simulink model "ES105A_StHlthSigNormn"  (R2013b)
settings: Solver=FixedStepDiscrete  SolverMode=SingleTasking  StartTime=0.0  StopTime=1  FixedStep=0.002  RelTol=1e-3
undefined symbols (not defined in the file): ARCHGLBPRM_FLOATZEROTHD_ULS_F32, CurrMeasCorrlnMaxErrCurr, CURRMOTSUMDIVBYZEROPROTNVAL_AMPR_F32, DIGTQDIVBYZEROPROTNVAL_HWNWTMTR_F32, DutyCycThermProtnDutyCycFildThd, EcuTMeasRngDiagcMax, EcuTMeasRngDiagcMin, EotLrngAuthyStrtLrn, FRICESTIMNDIVBYZEROPROTNVAL_HWNWTMTR_F32, HLTH0PERC_CNT_U08, HLTH100PERC_CNT_F32, HLTH100PERC_CNT_U08, HLTH50PERC_CNT_U08, HwTqCorrlnChATraSumSetFltThd, HwTqCorrlnChBTraSumSetFltThd, HWTQIDPTSIG_CNT_U08, MOTAG2MEAS_VALMAXERR_VOLTSQD_F32, MOTAG2MEAS_VALMINERR_VOLTSQD_F32, MOTAGCORRLN_MOTAGCORRLNERRTHD_MOTREVELEC_U0P16, MotDrvDiagcErrThd, MOTPOS2DIVBYZEROPROTNVAL2_VOLTSQD_F32, MOTPOS2DIVBYZEROPROTNVAL_VOLTSQD_F32, MOTPOSNERRDIVBYZEROPROTNVAL_MOTREV_U16, MOTPOSNERRZEROTHD_MOTREV_U0P16, NtcNr1, NtcSts1, PHAVLTGDIVBYZEROPROTNVAL_NANOSEC_F32, SigQlfr1, STHLTHSCAGFAC_CNT_F32, StHlthSigNormnAbsltMotPosDifStHlthDiagThd, StHlthSigNormnCurrMotSumStHlthDiagThd, StHlthSigNormnDigTqStHlthDiagThd, StHlthSigNormnDutyCycFltLimThd, StHlthSigNormnHiCtrlrT, StHlthSigNormnIdptSigStHlthSca, StHlthSigNormnLoCtrlrT, StHlthSigNormnMaxFricThd, StHlthSigNormnMinRackTrvlLim, StHlthSigNormnMotPosStHlthDiagThd, StHlthSigNormnMotVelCal, StHlthSigNormnPhaInfoStHlthDiagThd, StHlthSigNormnStHlthCorrlnErr, StHlthSigNormnStHlthCurrMotSum, StHlthSigNormnStHlthPhaInfo, StHlthSigNormnValMaxStHlthErr, StHlthSigNormnValMinStHlthErr, StHlthSigNormnWhlImbRejctnThd, SysGlbPrmMotPoleCnt, TSTHLTH0PERC_CNT_U08, u2, u3, u4, VLTGSTHLTH0PERC_CNT_U08
libraries: NxtrLim x39, simulink x33, NxtrAbslt x4
(part 9 of 10)

== system ES105A_StHlthSigNormn/StHlthSigNormn/UpdRawSig/Digital Torque Sensor /DigTqSnsrBStHlth Calc/If Action Subsystem3/Devide by Zero Protection for Cal/If Zero ==
  Action Port : ActionPort  ActionType=then
  Constant1 : Constant  Value=DIGTQDIVBYZEROPROTNVAL_HWNWTMTR_F32
  CopyRight2 : Subsystem  Description=|  mask(Copyright Information){none=on}
      | Copyright info block.                                               
      |                                                                     
      | Place copyright information at the top of every subsystem in design.
      mask prompts: none "No parameters"
      mask help: Place copyright information at the top of every subsystem in design.
      mask Display:
      | NxtrConf = 'Nexteer Confidential';
      | 
      | sys = bdroot; %handle for the current model ("system")
      | first = get_param(sys,'Created');
      | first = first(end-3:end);  %year is last four digits
      | 
      | last = get_param(sys,'LastModifiedDate');
      | if isempty(last)
      |     last = datestr(now,'yyyy');
      | else
      |     last = last(end-3:end);
      | end
      | 
      | if strcmp(first,last)
      |     fprintf('%s -- Copyright %s Nexteer',NxtrConf,first)
      | else
      |     fprintf('%s -- %s%s- %s Nexteer',NxtrConf,char(169),first,last)
      | end
  Out1 : Outport
  wires:
  Constant1/1 -> Out1/1

== system ES105A_StHlthSigNormn/StHlthSigNormn/UpdRawSig/Digital Torque Sensor /DigTqSnsrBStHlth Calc/If Action Subsystem3/Devide by Zero Protection for Cal/Non Zero ==
  In1 : Inport
  Action Port : ActionPort  ActionType=else
  CopyRight2 : Subsystem  Description=|  mask(Copyright Information){none=on}
      | Copyright info block.                                               
      |                                                                     
      | Place copyright information at the top of every subsystem in design.
      mask prompts: none "No parameters"
      mask help: Place copyright information at the top of every subsystem in design.
      mask Display:
      | NxtrConf = 'Nexteer Confidential';
      | 
      | sys = bdroot; %handle for the current model ("system")
      | first = get_param(sys,'Created');
      | first = first(end-3:end);  %year is last four digits
      | 
      | last = get_param(sys,'LastModifiedDate');
      | if isempty(last)
      |     last = datestr(now,'yyyy');
      | else
      |     last = last(end-3:end);
      | end
      | 
      | if strcmp(first,last)
      |     fprintf('%s -- Copyright %s Nexteer',NxtrConf,first)
      | else
      |     fprintf('%s -- %s%s- %s Nexteer',NxtrConf,char(169),first,last)
      | end
  Out1 : Outport
  wires:
  In1/1 -> Out1/1

== system ES105A_StHlthSigNormn/StHlthSigNormn/UpdRawSig/Friction Estimation/If Action Subsystem4/Divide by Zero Protection for Cal/If Zero/CopyRight2 ==

== system ES105A_StHlthSigNormn/StHlthSigNormn/UpdRawSig/Friction Estimation/If Action Subsystem4/Divide by Zero Protection for Cal/Non Zero/CopyRight2 ==

== system ES105A_StHlthSigNormn/StHlthSigNormn/UpdRawSig/Motor Position 2 /If Action Subsystem/If Action Subsystem1/Divide by Zero Protection for Cal/CopyRight2 ==

== system ES105A_StHlthSigNormn/StHlthSigNormn/UpdRawSig/Motor Position 2 /If Action Subsystem/If Action Subsystem1/Divide by Zero Protection for Cal/If Zero ==
  Action Port : ActionPort  ActionType=then
  Constant : Constant  Value=MOTPOS2DIVBYZEROPROTNVAL2_VOLTSQD_F32
  CopyRight2 : Subsystem  Description=|  mask(Copyright Information){none=on}
      | Copyright info block.                                               
      |                                                                     
      | Place copyright information at the top of every subsystem in design.
      mask prompts: none "No parameters"
      mask help: Place copyright information at the top of every subsystem in design.
      mask Display:
      | NxtrConf = 'Nexteer Confidential';
      | 
      | sys = bdroot; %handle for the current model ("system")
      | first = get_param(sys,'Created');
      | first = first(end-3:end);  %year is last four digits
      | 
      | last = get_param(sys,'LastModifiedDate');
      | if isempty(last)
      |     last = datestr(now,'yyyy');
      | else
      |     last = last(end-3:end);
      | end
      | 
      | if strcmp(first,last)
      |     fprintf('%s -- Copyright %s Nexteer',NxtrConf,first)
      | else
      |     fprintf('%s -- %s%s- %s Nexteer',NxtrConf,char(169),first,last)
      | end
  Out1 : Outport
  wires:
  Constant/1 -> Out1/1

== system ES105A_StHlthSigNormn/StHlthSigNormn/UpdRawSig/Motor Position 2 /If Action Subsystem/If Action Subsystem1/Divide by Zero Protection for Cal/Non Zero ==
  In1 : Inport
  Action Port : ActionPort  ActionType=else
  CopyRight2 : Subsystem  Description=|  mask(Copyright Information){none=on}
      | Copyright info block.                                               
      |                                                                     
      | Place copyright information at the top of every subsystem in design.
      mask prompts: none "No parameters"
      mask help: Place copyright information at the top of every subsystem in design.
      mask Display:
      | NxtrConf = 'Nexteer Confidential';
      | 
      | sys = bdroot; %handle for the current model ("system")
      | first = get_param(sys,'Created');
      | first = first(end-3:end);  %year is last four digits
      | 
      | last = get_param(sys,'LastModifiedDate');
      | if isempty(last)
      |     last = datestr(now,'yyyy');
      | else
      |     last = last(end-3:end);
      | end
      | 
      | if strcmp(first,last)
      |     fprintf('%s -- Copyright %s Nexteer',NxtrConf,first)
      | else
      |     fprintf('%s -- %s%s- %s Nexteer',NxtrConf,char(169),first,last)
      | end
  Out1 : Outport
  wires:
  In1/1 -> Out1/1

== system ES105A_StHlthSigNormn/StHlthSigNormn/UpdRawSig/Motor Position 2 /If Action Subsystem/If Action Subsystem2/Divide by Zero Protection for Cal/CopyRight2 ==

== system ES105A_StHlthSigNormn/StHlthSigNormn/UpdRawSig/Motor Position 2 /If Action Subsystem/If Action Subsystem2/Divide by Zero Protection for Cal/If Zero ==
  Action Port : ActionPort  ActionType=then
  Constant : Constant  Value=MOTPOS2DIVBYZEROPROTNVAL_VOLTSQD_F32
  CopyRight2 : Subsystem  Description=|  mask(Copyright Information){none=on}
      | Copyright info block.                                               
      |                                                                     
      | Place copyright information at the top of every subsystem in design.
      mask prompts: none "No parameters"
      mask help: Place copyright information at the top of every subsystem in design.
      mask Display:
      | NxtrConf = 'Nexteer Confidential';
      | 
      | sys = bdroot; %handle for the current model ("system")
      | first = get_param(sys,'Created');
      | first = first(end-3:end);  %year is last four digits
      | 
      | last = get_param(sys,'LastModifiedDate');
      | if isempty(last)
      |     last = datestr(now,'yyyy');
      | else
      |     last = last(end-3:end);
      | end
      | 
      | if strcmp(first,last)
      |     fprintf('%s -- Copyright %s Nexteer',NxtrConf,first)
      | else
      |     fprintf('%s -- %s%s- %s Nexteer',NxtrConf,char(169),first,last)
      | end
  Out1 : Outport
  wires:
  Constant/1 -> Out1/1

== system ES105A_StHlthSigNormn/StHlthSigNormn/UpdRawSig/Motor Position 2 /If Action Subsystem/If Action Subsystem2/Divide by Zero Protection for Cal/Non Zero ==
  In1 : Inport
  Action Port : ActionPort  ActionType=else
  CopyRight2 : Subsystem  Description=|  mask(Copyright Information){none=on}
      | Copyright info block.                                               
      |                                                                     
      | Place copyright information at the top of every subsystem in design.
      mask prompts: none "No parameters"
      mask help: Place copyright information at the top of every subsystem in design.
      mask Display:
      | NxtrConf = 'Nexteer Confidential';
      | 
      | sys = bdroot; %handle for the current model ("system")
      | first = get_param(sys,'Created');
      | first = first(end-3:end);  %year is last four digits
      | 
      | last = get_param(sys,'LastModifiedDate');
      | if isempty(last)
      |     last = datestr(now,'yyyy');
      | else
      |     last = last(end-3:end);
      | end
      | 
      | if strcmp(first,last)
      |     fprintf('%s -- Copyright %s Nexteer',NxtrConf,first)
      | else
      |     fprintf('%s -- %s%s- %s Nexteer',NxtrConf,char(169),first,last)
      | end
  Out1 : Outport
  wires:
  In1/1 -> Out1/1

== system ES105A_StHlthSigNormn/StHlthSigNormn/UpdRawSig/Motor Position Error /AbsltMotPosABDifStHlth Calc/If Action Subsystem/If Action Subsystem/CopyRight2 ==

== system ES105A_StHlthSigNormn/StHlthSigNormn/UpdRawSig/Motor Position Error /AbsltMotPosABDifStHlth Calc/If Action Subsystem/If Action Subsystem1/CopyRight2 ==

== system ES105A_StHlthSigNormn/StHlthSigNormn/UpdRawSig/Motor Position Error /AbsltMotPosABDifStHlth Calc/If Action Subsystem/If Action Subsystem1/Divide by Zero Protection for Cal ==
  Constant : Constant  Value=MOTPOSNERRZEROTHD_MOTREV_U0P16  OutDataTypeStr=uint16
      settings: AttributesFormatString=%<OutDataTypeStr>
  Constant2 : Constant  Value=StHlthSigNormnStHlthCorrlnErr
  CopyRight2 : Subsystem  Description=|  mask(Copyright Information){none=on}
      | Copyright info block.                                               
      |                                                                     
      | Place copyright information at the top of every subsystem in design.
      mask prompts: none "No parameters"
      mask help: Place copyright information at the top of every subsystem in design.
      mask Display:
      | NxtrConf = 'Nexteer Confidential';
      | 
      | sys = bdroot; %handle for the current model ("system")
      | first = get_param(sys,'Created');
      | first = first(end-3:end);  %year is last four digits
      | 
      | last = get_param(sys,'LastModifiedDate');
      | if isempty(last)
      |     last = datestr(now,'yyyy');
      | else
      |     last = last(end-3:end);
      | end
      | 
      | if strcmp(first,last)
      |     fprintf('%s -- Copyright %s Nexteer',NxtrConf,first)
      | else
      |     fprintf('%s -- %s%s- %s Nexteer',NxtrConf,char(169),first,last)
      | end
  Data Store Read1 : DataStoreRead  DataStoreName=MotAgCorrlnErrThd
  If : If  IfExpression=u1
  If Zero : Subsystem  TreatAsAtomicUnit=on
  Merge : Merge
  Non Zero : Subsystem  TreatAsAtomicUnit=on
  Relational Operator : RelationalOperator  Operator=<=  OutDataTypeStr=boolean
  Subtract2 : Sum  Inputs=+-
  CorrlnDelta : Outport
  wires:
  If/1 -> If Zero/Action
  If/2 -> Non Zero/Action
  If Zero/1(Out1) -> Merge/1
  Non Zero/1(Out1) -> Merge/2
  Merge/1 -> CorrlnDelta/1
  Relational Operator/1 -> If/1
  Constant/1 -> Relational Operator/2
  Constant2/1 -> Subtract2/2
  Data Store Read1/1 -> Subtract2/1
  Subtract2/1 -> Non Zero/1(In1), Relational Operator/1

== system ES105A_StHlthSigNormn/StHlthSigNormn/UpdRawSig/Motor Position Error /AbsltMotPosACDifStHlth Calc/If Action Subsystem4/If Action Subsystem/CopyRight2 ==

== system ES105A_StHlthSigNormn/StHlthSigNormn/UpdRawSig/Motor Position Error /AbsltMotPosACDifStHlth Calc/If Action Subsystem4/If Action Subsystem1/CopyRight2 ==

== system ES105A_StHlthSigNormn/StHlthSigNormn/UpdRawSig/Motor Position Error /AbsltMotPosACDifStHlth Calc/If Action Subsystem4/If Action Subsystem1/Divide by Zero Protection for Cal ==
  Constant1 : Constant  Value=MOTPOSNERRZEROTHD_MOTREV_U0P16  OutDataTypeStr=uint16
      settings: AttributesFormatString=%<OutDataTypeStr>
  Constant2 : Constant  Value=StHlthSigNormnStHlthCorrlnErr
  CopyRight2 : Subsystem  Description=|  mask(Copyright Information){none=on}
      | Copyright info block.                                               
      |                                                                     
      | Place copyright information at the top of every subsystem in design.
      mask prompts: none "No parameters"
      mask help: Place copyright information at the top of every subsystem in design.
      mask Display:
      | NxtrConf = 'Nexteer Confidential';
      | 
      | sys = bdroot; %handle for the current model ("system")
      | first = get_param(sys,'Created');
      | first = first(end-3:end);  %year is last four digits
      | 
      | last = get_param(sys,'LastModifiedDate');
      | if isempty(last)
      |     last = datestr(now,'yyyy');
      | else
      |     last = last(end-3:end);
      | end
      | 
      | if strcmp(first,last)
      |     fprintf('%s -- Copyright %s Nexteer',NxtrConf,first)
      | else
      |     fprintf('%s -- %s%s- %s Nexteer',NxtrConf,char(169),first,last)
      | end
  Data Store Read1 : DataStoreRead  DataStoreName=MotAgCorrlnErrThd
  If : If  IfExpression=u1
  If Zero : Subsystem  TreatAsAtomicUnit=on
  Merge : Merge
  Non Zero : Subsystem  TreatAsAtomicUnit=on
  Relational Operator : RelationalOperator  Operator=<=  OutDataTypeStr=boolean
  Subtract2 : Sum  Inputs=+-
  CorrlnDelta : Outport
  wires:
  If/1 -> If Zero/Action
  If/2 -> Non Zero/Action
  If Zero/1(Out1) -> Merge/1
  Non Zero/1(Out1) -> Merge/2
  Merge/1 -> CorrlnDelta/1
  Relational Operator/1 -> If/1
  Constant1/1 -> Relational Operator/2
  Constant2/1 -> Subtract2/2
  Data Store Read1/1 -> Subtract2/1
  Subtract2/1 -> Relational Operator/1, Non Zero/1(In1)

== system ES105A_StHlthSigNormn/StHlthSigNormn/UpdRawSig/Motor Position Error /AbsltMotPosBCDifStHlth Calc/If Action Subsystem8/If Action Subsystem/CopyRight2 ==

== system ES105A_StHlthSigNormn/StHlthSigNormn/UpdRawSig/Motor Position Error /AbsltMotPosBCDifStHlth Calc/If Action Subsystem8/If Action Subsystem1/CopyRight2 ==

== system ES105A_StHlthSigNormn/StHlthSigNormn/UpdRawSig/Motor Position Error /AbsltMotPosBCDifStHlth Calc/If Action Subsystem8/If Action Subsystem1/Divide by Zero Protection for Cal ==
  Constant1 : Constant  Value=MOTPOSNERRZEROTHD_MOTREV_U0P16  OutDataTypeStr=uint16
      settings: AttributesFormatString=%<OutDataTypeStr>
  Constant2 : Constant  Value=StHlthSigNormnStHlthCorrlnErr
  CopyRight2 : Subsystem  Description=|  mask(Copyright Information){none=on}
      | Copyright info block.                                               
      |                                                                     
      | Place copyright information at the top of every subsystem in design.
      mask prompts: none "No parameters"
      mask help: Place copyright information at the top of every subsystem in design.
      mask Display:
      | NxtrConf = 'Nexteer Confidential';
      | 
      | sys = bdroot; %handle for the current model ("system")
      | first = get_param(sys,'Created');
      | first = first(end-3:end);  %year is last four digits
      | 
      | last = get_param(sys,'LastModifiedDate');
      | if isempty(last)
      |     last = datestr(now,'yyyy');
      | else
      |     last = last(end-3:end);
      | end
      | 
      | if strcmp(first,last)
      |     fprintf('%s -- Copyright %s Nexteer',NxtrConf,first)
      | else
      |     fprintf('%s -- %s%s- %s Nexteer',NxtrConf,char(169),first,last)
      | end
  Data Store Read1 : DataStoreRead  DataStoreName=MotAgCorrlnErrThd
  If : If  IfExpression=u1
  If Zero : Subsystem  TreatAsAtomicUnit=on
  Merge : Merge
  Non Zero : Subsystem  TreatAsAtomicUnit=on
  Relational Operator : RelationalOperator  Operator=<=  OutDataTypeStr=boolean
  Subtract2 : Sum  Inputs=+-
  CorrlnDelta : Outport
  wires:
  If/1 -> If Zero/Action
  If/2 -> Non Zero/Action
  If Zero/1(Out1) -> Merge/1
  Non Zero/1(Out1) -> Merge/2
  Merge/1 -> CorrlnDelta/1
  Relational Operator/1 -> If/1
  Constant1/1 -> Relational Operator/2
  Constant2/1 -> Subtract2/2
  Data Store Read1/1 -> Subtract2/1
  Subtract2/1 -> Non Zero/1(In1), Relational Operator/1

== system ES105A_StHlthSigNormn/StHlthSigNormn/UpdRawSig/Phase Voltage Verification/PhaAStHlth Calc/If Action Subsystem/If Action Subsystem/CopyRight2 ==

== system ES105A_StHlthSigNormn/StHlthSigNormn/UpdRawSig/Phase Voltage Verification/PhaAStHlth Calc/If Action Subsystem/If Action Subsystem1/CopyRight2 ==

== system ES105A_StHlthSigNormn/StHlthSigNormn/UpdRawSig/Phase Voltage Verification/PhaAStHlth Calc/If Action Subsystem/If Action Subsystem1/Divide by Zero Protection for Cal ==
  Compare To Zero : simulink/Logic and Bit Operations/Compare To Zero  relop===  OutDataTypeStr=boolean
  Constant2 : Constant  Value=StHlthSigNormnStHlthPhaInfo
  Constant4 : Constant  Value=MotDrvDiagcErrThd
  CopyRight2 : Subsystem  Description=|  mask(Copyright Information){none=on}
      | Copyright info block.                                               
      |                                                                     
      | Place copyright information at the top of every subsystem in design.
      mask prompts: none "No parameters"
      mask help: Place copyright information at the top of every subsystem in design.
      mask Display:
      | NxtrConf = 'Nexteer Confidential';
      | 
      | sys = bdroot; %handle for the current model ("system")
      | first = get_param(sys,'Created');
      | first = first(end-3:end);  %year is last four digits
      | 
      | last = get_param(sys,'LastModifiedDate');
      | if isempty(last)
      |     last = datestr(now,'yyyy');
      | else
      |     last = last(end-3:end);
      | end
      | 
      | if strcmp(first,last)
      |     fprintf('%s -- Copyright %s Nexteer',NxtrConf,first)
      | else
      |     fprintf('%s -- %s%s- %s Nexteer',NxtrConf,char(169),first,last)
      | end
  If : If  IfExpression=u1
  If Zero : Subsystem  TreatAsAtomicUnit=on
  Merge : Merge
  Non Zero : Subsystem  TreatAsAtomicUnit=on
  Subtract2 : Sum  Inputs=+-
  MotDrvDiagDelta : Outport
  wires:
  If/1 -> If Zero/Action
  If/2 -> Non Zero/Action
  If Zero/1(Out1) -> Merge/1
  Non Zero/1(Out1) -> Merge/2
  Merge/1 -> MotDrvDiagDelta/1
  Subtract2/1 -> Non Zero/1(In1), Compare To Zero/1
  Constant4/1 -> Subtract2/1
  Constant2/1 -> Subtract2/2
  Compare To Zero/1 -> If/1

== system ES105A_StHlthSigNormn/StHlthSigNormn/UpdRawSig/Phase Voltage Verification/PhaBStHlth Calc/If Action Subsystem4/If Action Subsystem/CopyRight2 ==

== system ES105A_StHlthSigNormn/StHlthSigNormn/UpdRawSig/Phase Voltage Verification/PhaBStHlth Calc/If Action Subsystem4/If Action Subsystem1/CopyRight2 ==

== system ES105A_StHlthSigNormn/StHlthSigNormn/UpdRawSig/Phase Voltage Verification/PhaBStHlth Calc/If Action Subsystem4/If Action Subsystem1/Divide by Zero Protection for Cal ==
  Compare To Zero : simulink/Logic and Bit Operations/Compare To Zero  relop===  OutDataTypeStr=boolean
  Constant2 : Constant  Value=StHlthSigNormnStHlthPhaInfo
  Constant4 : Constant  Value=MotDrvDiagcErrThd
  CopyRight2 : Subsystem  Description=|  mask(Copyright Information){none=on}
      | Copyright info block.                                               
      |                                                                     
      | Place copyright information at the top of every subsystem in design.
      mask prompts: none "No parameters"
      mask help: Place copyright information at the top of every subsystem in design.
      mask Display:
      | NxtrConf = 'Nexteer Confidential';
      | 
      | sys = bdroot; %handle for the current model ("system")
      | first = get_param(sys,'Created');
      | first = first(end-3:end);  %year is last four digits
      | 
      | last = get_param(sys,'LastModifiedDate');
      | if isempty(last)
      |     last = datestr(now,'yyyy');
      | else
      |     last = last(end-3:end);
      | end
      | 
      | if strcmp(first,last)
      |     fprintf('%s -- Copyright %s Nexteer',NxtrConf,first)
      | else
      |     fprintf('%s -- %s%s- %s Nexteer',NxtrConf,char(169),first,last)
      | end
  If : If  IfExpression=u1
  If Zero : Subsystem  TreatAsAtomicUnit=on
  Merge : Merge
  Non Zero : Subsystem  TreatAsAtomicUnit=on
  Subtract2 : Sum  Inputs=+-
  MotDrvDiagDelta : Outport
  wires:
  If/1 -> If Zero/Action
  If/2 -> Non Zero/Action
  If Zero/1(Out1) -> Merge/1
  Non Zero/1(Out1) -> Merge/2
  Merge/1 -> MotDrvDiagDelta/1
  Subtract2/1 -> Non Zero/1(In1), Compare To Zero/1
  Constant4/1 -> Subtract2/1
  Constant2/1 -> Subtract2/2
  Compare To Zero/1 -> If/1

== system ES105A_StHlthSigNormn/StHlthSigNormn/UpdRawSig/Phase Voltage Verification/PhaCStHlth Calc/If Action Subsystem8/If Action Subsystem/CopyRight2 ==

== system ES105A_StHlthSigNormn/StHlthSigNormn/UpdRawSig/Phase Voltage Verification/PhaCStHlth Calc/If Action Subsystem8/If Action Subsystem1/CopyRight2 ==

== system ES105A_StHlthSigNormn/StHlthSigNormn/UpdRawSig/Phase Voltage Verification/PhaCStHlth Calc/If Action Subsystem8/If Action Subsystem1/Divide by Zero Protection for Cal ==
  Compare To Zero : simulink/Logic and Bit Operations/Compare To Zero  relop===  OutDataTypeStr=boolean
  Constant2 : Constant  Value=StHlthSigNormnStHlthPhaInfo
  Constant4 : Constant  Value=MotDrvDiagcErrThd
  CopyRight2 : Subsystem  Description=|  mask(Copyright Information){none=on}
      | Copyright info block.                                               
      |                                                                     
      | Place copyright information at the top of every subsystem in design.
      mask prompts: none "No parameters"
      mask help: Place copyright information at the top of every subsystem in design.
      mask Display:
      | NxtrConf = 'Nexteer Confidential';
      | 
      | sys = bdroot; %handle for the current model ("system")
      | first = get_param(sys,'Created');
      | first = first(end-3:end);  %year is last four digits
      | 
      | last = get_param(sys,'LastModifiedDate');
      | if isempty(last)
      |     last = datestr(now,'yyyy');
      | else
      |     last = last(end-3:end);
      | end
      | 
      | if strcmp(first,last)
      |     fprintf('%s -- Copyright %s Nexteer',NxtrConf,first)
      | else
      |     fprintf('%s -- %s%s- %s Nexteer',NxtrConf,char(169),first,last)
      | end
  If : If  IfExpression=u1
  If Zero : Subsystem  TreatAsAtomicUnit=on
  Merge : Merge
  Non Zero : Subsystem  TreatAsAtomicUnit=on
  Subtract2 : Sum  Inputs=+-
  MotDrvDiagDelta : Outport
  wires:
  If/1 -> If Zero/Action
  If/2 -> Non Zero/Action
  If Zero/1(Out1) -> Merge/1
  Non Zero/1(Out1) -> Merge/2
  Merge/1 -> MotDrvDiagDelta/1
  Subtract2/1 -> Non Zero/1(In1), Compare To Zero/1
  Constant4/1 -> Subtract2/1
  Constant2/1 -> Subtract2/2
  Compare To Zero/1 -> If/1

== system ES105A_StHlthSigNormn/StHlthSigNormn/UpdRawSig/Phase Voltage Verification/PhaDStHlth Calc/If Action Subsystem12/If Action Subsystem/CopyRight2 ==

== system ES105A_StHlthSigNormn/StHlthSigNormn/UpdRawSig/Phase Voltage Verification/PhaDStHlth Calc/If Action Subsystem12/If Action Subsystem1/CopyRight2 ==

== system ES105A_StHlthSigNormn/StHlthSigNormn/UpdRawSig/Phase Voltage Verification/PhaDStHlth Calc/If Action Subsystem12/If Action Subsystem1/Divide by Zero Protection for Cal ==
  Compare To Zero : simulink/Logic and Bit Operations/Compare To Zero  relop===  OutDataTypeStr=boolean
  Constant2 : Constant  Value=StHlthSigNormnStHlthPhaInfo
  Constant4 : Constant  Value=MotDrvDiagcErrThd
  CopyRight2 : Subsystem  Description=|  mask(Copyright Information){none=on}
      | Copyright info block.                                               
      |                                                                     
      | Place copyright information at the top of every subsystem in design.
      mask prompts: none "No parameters"
      mask help: Place copyright information at the top of every subsystem in design.
      mask Display:
      | NxtrConf = 'Nexteer Confidential';
      | 
      | sys = bdroot; %handle for the current model ("system")
      | first = get_param(sys,'Created');
      | first = first(end-3:end);  %year is last four digits
      | 
      | last = get_param(sys,'LastModifiedDate');
      | if isempty(last)
      |     last = datestr(now,'yyyy');
      | else
      |     last = last(end-3:end);
      | end
      | 
      | if strcmp(first,last)
      |     fprintf('%s -- Copyright %s Nexteer',NxtrConf,first)
      | else
      |     fprintf('%s -- %s%s- %s Nexteer',NxtrConf,char(169),first,last)
      | end
  If : If  IfExpression=u1
  If Zero : Subsystem  TreatAsAtomicUnit=on
  Merge : Merge
  Non Zero : Subsystem  TreatAsAtomicUnit=on
  Subtract2 : Sum  Inputs=+-
  MotDrvDiagDelta : Outport
  wires:
  If/1 -> If Zero/Action
  If/2 -> Non Zero/Action
  If Zero/1(Out1) -> Merge/1
  Non Zero/1(Out1) -> Merge/2
  Merge/1 -> MotDrvDiagDelta/1
  Subtract2/1 -> Non Zero/1(In1), Compare To Zero/1
  Constant4/1 -> Subtract2/1
  Constant2/1 -> Subtract2/2
  Compare To Zero/1 -> If/1

== system ES105A_StHlthSigNormn/StHlthSigNormn/UpdRawSig/Phase Voltage Verification/PhaEStHlth Calc/If Action Subsystem16/If Action Subsystem/CopyRight2 ==

== system ES105A_StHlthSigNormn/StHlthSigNormn/UpdRawSig/Phase Voltage Verification/PhaEStHlth Calc/If Action Subsystem16/If Action Subsystem1/CopyRight2 ==

== system ES105A_StHlthSigNormn/StHlthSigNormn/UpdRawSig/Phase Voltage Verification/PhaEStHlth Calc/If Action Subsystem16/If Action Subsystem1/Divide by Zero Protection for Cal ==
  Compare To Zero : simulink/Logic and Bit Operations/Compare To Zero  relop===  OutDataTypeStr=boolean
  Constant2 : Constant  Value=StHlthSigNormnStHlthPhaInfo
  Constant4 : Constant  Value=MotDrvDiagcErrThd
  CopyRight2 : Subsystem  Description=|  mask(Copyright Information){none=on}
      | Copyright info block.                                               
      |                                                                     
      | Place copyright information at the top of every subsystem in design.
      mask prompts: none "No parameters"
      mask help: Place copyright information at the top of every subsystem in design.
      mask Display:
      | NxtrConf = 'Nexteer Confidential';
      | 
      | sys = bdroot; %handle for the current model ("system")
      | first = get_param(sys,'Created');
      | first = first(end-3:end);  %year is last four digits
      | 
      | last = get_param(sys,'LastModifiedDate');
      | if isempty(last)
      |     last = datestr(now,'yyyy');
      | else
      |     last = last(end-3:end);
      | end
      | 
      | if strcmp(first,last)
      |     fprintf('%s -- Copyright %s Nexteer',NxtrConf,first)
      | else
      |     fprintf('%s -- %s%s- %s Nexteer',NxtrConf,char(169),first,last)
      | end
  If : If  IfExpression=u1
  If Zero : Subsystem  TreatAsAtomicUnit=on
  Merge : Merge
  Non Zero : Subsystem  TreatAsAtomicUnit=on
  Subtract2 : Sum  Inputs=+-
  MotDrvDiagDelta : Outport
  wires:
  If/1 -> If Zero/Action
  If/2 -> Non Zero/Action
  If Zero/1(Out1) -> Merge/1
  Non Zero/1(Out1) -> Merge/2
  Merge/1 -> MotDrvDiagDelta/1
  Subtract2/1 -> Non Zero/1(In1), Compare To Zero/1
  Constant4/1 -> Subtract2/1
  Constant2/1 -> Subtract2/2
  Compare To Zero/1 -> If/1

== system ES105A_StHlthSigNormn/StHlthSigNormn/UpdRawSig/Phase Voltage Verification/PhaFStHlth Calc/If Action Subsystem20/If Action Subsystem/CopyRight2 ==

== system ES105A_StHlthSigNormn/StHlthSigNormn/UpdRawSig/Phase Voltage Verification/PhaFStHlth Calc/If Action Subsystem20/If Action Subsystem1/CopyRight2 ==

== system ES105A_StHlthSigNormn/StHlthSigNormn/UpdRawSig/Phase Voltage Verification/PhaFStHlth Calc/If Action Subsystem20/If Action Subsystem1/Divide by Zero Protection for Cal ==
  Compare To Zero : simulink/Logic and Bit Operations/Compare To Zero  relop===  OutDataTypeStr=boolean
  Constant2 : Constant  Value=StHlthSigNormnStHlthPhaInfo
  Constant4 : Constant  Value=MotDrvDiagcErrThd
  CopyRight2 : Subsystem  Description=|  mask(Copyright Information){none=on}
      | Copyright info block.                                               
      |                                                                     
      | Place copyright information at the top of every subsystem in design.
      mask prompts: none "No parameters"
      mask help: Place copyright information at the top of every subsystem in design.
      mask Display:
      | NxtrConf = 'Nexteer Confidential';
      | 
      | sys = bdroot; %handle for the current model ("system")
      | first = get_param(sys,'Created');
      | first = first(end-3:end);  %year is last four digits
      | 
      | last = get_param(sys,'LastModifiedDate');
      | if isempty(last)
      |     last = datestr(now,'yyyy');
      | else
      |     last = last(end-3:end);
      | end
      | 
      | if strcmp(first,last)
      |     fprintf('%s -- Copyright %s Nexteer',NxtrConf,first)
      | else
      |     fprintf('%s -- %s%s- %s Nexteer',NxtrConf,char(169),first,last)
      | end
  If : If  IfExpression=u1
  If Zero : Subsystem  TreatAsAtomicUnit=on
  Merge : Merge
  Non Zero : Subsystem  TreatAsAtomicUnit=on
  Subtract2 : Sum  Inputs=+-
  MotDrvDiagDelta : Outport
  wires:
  If/1 -> If Zero/Action
  If/2 -> Non Zero/Action
  If Zero/1(Out1) -> Merge/1
  Non Zero/1(Out1) -> Merge/2
  Merge/1 -> MotDrvDiagDelta/1
  Subtract2/1 -> Non Zero/1(In1), Compare To Zero/1
  Constant4/1 -> Subtract2/1
  Constant2/1 -> Subtract2/2
  Compare To Zero/1 -> If/1

== system ES105A_StHlthSigNormn/StHlthSigNormn/UpdRawSig/ EOT Impact Counter/If Action Subsystem/If Action Subsystem/If Action Subsystem/Do nothing/CopyRight2 ==

== system ES105A_StHlthSigNormn/StHlthSigNormn/UpdRawSig/ EOT Impact Counter/If Action Subsystem/If Action Subsystem/If Action Subsystem/If Action Subsystem/CopyRight2 ==

== system ES105A_StHlthSigNormn/StHlthSigNormn/UpdRawSig/ EOT Impact Counter/If Action Subsystem/If Action Subsystem/If Action Subsystem/If Action Subsystem/Do Nothing ==
  note: Do Nothing
  Action Port : ActionPort  ActionType=else
  CopyRight2 : Subsystem  Description=|  mask(Copyright Information){none=on}
      | Copyright info block.                                               
      |                                                                     
      | Place copyright information at the top of every subsystem in design.
      mask prompts: none "No parameters"
      mask help: Place copyright information at the top of every subsystem in design.
      mask Display:
      | NxtrConf = 'Nexteer Confidential';
      | 
      | sys = bdroot; %handle for the current model ("system")
      | first = get_param(sys,'Created');
      | first = first(end-3:end);  %year is last four digits
      | 
      | last = get_param(sys,'LastModifiedDate');
      | if isempty(last)
      |     last = datestr(now,'yyyy');
      | else
      |     last = last(end-3:end);
      | end
      | 
      | if strcmp(first,last)
      |     fprintf('%s -- Copyright %s Nexteer',NxtrConf,first)
      | else
      |     fprintf('%s -- %s%s- %s Nexteer',NxtrConf,char(169),first,last)
      | end

== system ES105A_StHlthSigNormn/StHlthSigNormn/UpdRawSig/ EOT Impact Counter/If Action Subsystem/If Action Subsystem/If Action Subsystem/If Action Subsystem/If Action Subsystem ==
  Action Port : ActionPort  ActionType=then
  Constant : Constant  OutDataTypeStr=boolean
      settings: AttributesFormatString=%<OutDataTypeStr>
  Constant1 : Constant  Value=0  OutDataTypeStr=uint8
      settings: AttributesFormatString=%<OutDataTypeStr>
  CopyRight2 : Subsystem  Description=|  mask(Copyright Information){none=on}
      | Copyright info block.                                               
      |                                                                     
      | Place copyright information at the top of every subsystem in design.
      mask prompts: none "No parameters"
      mask help: Place copyright information at the top of every subsystem in design.
      mask Display:
      | NxtrConf = 'Nexteer Confidential';
      | 
      | sys = bdroot; %handle for the current model ("system")
      | first = get_param(sys,'Created');
      | first = first(end-3:end);  %year is last four digits
      | 
      | last = get_param(sys,'LastModifiedDate');
      | if isempty(last)
      |     last = datestr(now,'yyyy');
      | else
      |     last = last(end-3:end);
      | end
      | 
      | if strcmp(first,last)
      |     fprintf('%s -- Copyright %s Nexteer',NxtrConf,first)
      | else
      |     fprintf('%s -- %s%s- %s Nexteer',NxtrConf,char(169),first,last)
      | end
  Data Store Read : DataStoreRead  DataStoreName=EotImpctCntr
  Data Store Write : DataStoreWrite  DataStoreName=EntrEot
  Do nothing : Subsystem  TreatAsAtomicUnit=on
  If : If  IfExpression=u1
  If Action Subsystem : Subsystem  TreatAsAtomicUnit=on
  Relational Operator1 : RelationalOperator  Operator=>  OutDataTypeStr=boolean
  wires:
  Constant/1 -> Data Store Write/1
  Data Store Read/1 -> Relational Operator1/1
  Constant1/1 -> Relational Operator1/2
  Relational Operator1/1 -> If/1
  If/1 -> If Action Subsystem/Action
  If/2 -> Do nothing/Action

== system ES105A_StHlthSigNormn/StHlthSigNormn/UpdRawSig/ EOT Impact Counter/If Action Subsystem/If Action Subsystem1/If Action Subsystem/Do nothing/CopyRight2 ==

== system ES105A_StHlthSigNormn/StHlthSigNormn/UpdRawSig/ EOT Impact Counter/If Action Subsystem/If Action Subsystem1/If Action Subsystem/If Action Subsystem/CopyRight2 ==

== system ES105A_StHlthSigNormn/StHlthSigNormn/UpdRawSig/ EOT Impact Counter/If Action Subsystem/If Action Subsystem1/If Action Subsystem/If Action Subsystem/Do nothing ==
  note: Do Nothing
  Action Port : ActionPort  ActionType=else
  CopyRight2 : Subsystem  Description=|  mask(Copyright Information){none=on}
      | Copyright info block.                                               
      |                                                                     
      | Place copyright information at the top of every subsystem in design.
      mask prompts: none "No parameters"
      mask help: Place copyright information at the top of every subsystem in design.
      mask Display:
      | NxtrConf = 'Nexteer Confidential';
      | 
      | sys = bdroot; %handle for the current model ("system")
      | first = get_param(sys,'Created');
      | first = first(end-3:end);  %year is last four digits
      | 
      | last = get_param(sys,'LastModifiedDate');
      | if isempty(last)
      |     last = datestr(now,'yyyy');
      | else
      |     last = last(end-3:end);
      | end
      | 
      | if strcmp(first,last)
      |     fprintf('%s -- Copyright %s Nexteer',NxtrConf,first)
      | else
      |     fprintf('%s -- %s%s- %s Nexteer',NxtrConf,char(169),first,last)
      | end

== system ES105A_StHlthSigNormn/StHlthSigNormn/UpdRawSig/ EOT Impact Counter/If Action Subsystem/If Action Subsystem1/If Action Subsystem/If Action Subsystem/If Action Subsystem ==
  Action Port : ActionPort  ActionType=then
  Constant : Constant  OutDataTypeStr=boolean
      settings: AttributesFormatString=%<OutDataTypeStr>
  Constant1 : Constant  Value=0  OutDataTypeStr=uint8
      settings: AttributesFormatString=%<OutDataTypeStr>
  CopyRight2 : Subsystem  Description=|  mask(Copyright Information){none=on}
      | Copyright info block.                                               
      |                                                                     
      | Place copyright information at the top of every subsystem in design.
      mask prompts: none "No parameters"
      mask help: Place copyright information at the top of every subsystem in design.
      mask Display:
      | NxtrConf = 'Nexteer Confidential';
      | 
      | sys = bdroot; %handle for the current model ("system")
      | first = get_param(sys,'Created');
      | first = first(end-3:end);  %year is last four digits
      | 
      | last = get_param(sys,'LastModifiedDate');
      | if isempty(last)
      |     last = datestr(now,'yyyy');
      | else
      |     last = last(end-3:end);
      | end
      | 
      | if strcmp(first,last)
      |     fprintf('%s -- Copyright %s Nexteer',NxtrConf,first)
      | else
      |     fprintf('%s -- %s%s- %s Nexteer',NxtrConf,char(169),first,last)
      | end
  DO Nothing : Subsystem  TreatAsAtomicUnit=on
  Data Store Read : DataStoreRead  DataStoreName=EotImpctCntr
  Data Store Write : DataStoreWrite  DataStoreName=EntrEot
  If : If  IfExpression=u1
  If Action Subsystem : Subsystem  TreatAsAtomicUnit=on
  Relational Operator1 : RelationalOperator  Operator=>  OutDataTypeStr=boolean
  wires:
  Constant/1 -> Data Store Write/1
  Data Store Read/1 -> Relational Operator1/1
  Constant1/1 -> Relational Operator1/2
  Relational Operator1/1 -> If/1
  If/1 -> If Action Subsystem/Action
  If/2 -> DO Nothing/Action

== system ES105A_StHlthSigNormn/StHlthSigNormn/UpdRawSig/Current Error/CurrMotSumABCStHlth Calc/If Action Subsystem/If Action Subsystem1/Divide by Zero Protection for Cal/CopyRight2 ==

== system ES105A_StHlthSigNormn/StHlthSigNormn/UpdRawSig/Current Error/CurrMotSumABCStHlth Calc/If Action Subsystem/If Action Subsystem1/Divide by Zero Protection for Cal/If Zero ==
  Action Port : ActionPort  ActionType=then
  Constant : Constant  Value=CURRMOTSUMDIVBYZEROPROTNVAL_AMPR_F32
  CopyRight2 : Subsystem  Description=|  mask(Copyright Information){none=on}
      | Copyright info block.                                               
      |                                                                     
      | Place copyright information at the top of every subsystem in design.
      mask prompts: none "No parameters"
      mask help: Place copyright information at the top of every subsystem in design.
      mask Display:
      | NxtrConf = 'Nexteer Confidential';
      | 
      | sys = bdroot; %handle for the current model ("system")
      | first = get_param(sys,'Created');
      | first = first(end-3:end);  %year is last four digits
      | 
      | last = get_param(sys,'LastModifiedDate');
      | if isempty(last)
      |     last = datestr(now,'yyyy');
      | else
      |     last = last(end-3:end);
      | end
      | 
      | if strcmp(first,last)
      |     fprintf('%s -- Copyright %s Nexteer',NxtrConf,first)
      | else
      |     fprintf('%s -- %s%s- %s Nexteer',NxtrConf,char(169),first,last)
      | end
  Out1 : Outport
  wires:
  Constant/1 -> Out1/1

== system ES105A_StHlthSigNormn/StHlthSigNormn/UpdRawSig/Current Error/CurrMotSumABCStHlth Calc/If Action Subsystem/If Action Subsystem1/Divide by Zero Protection for Cal/Non Zero ==
  In1 : Inport
  Action Port : ActionPort  ActionType=else
  CopyRight2 : Subsystem  Description=|  mask(Copyright Information){none=on}
      | Copyright info block.                                               
      |                                                                     
      | Place copyright information at the top of every subsystem in design.
      mask prompts: none "No parameters"
      mask help: Place copyright information at the top of every subsystem in design.
      mask Display:
      | NxtrConf = 'Nexteer Confidential';
      | 
      | sys = bdroot; %handle for the current model ("system")
      | first = get_param(sys,'Created');
      | first = first(end-3:end);  %year is last four digits
      | 
      | last = get_param(sys,'LastModifiedDate');
      | if isempty(last)
      |     last = datestr(now,'yyyy');
      | else
      |     last = last(end-3:end);
      | end
      | 
      | if strcmp(first,last)
      |     fprintf('%s -- Copyright %s Nexteer',NxtrConf,first)
      | else
      |     fprintf('%s -- %s%s- %s Nexteer',NxtrConf,char(169),first,last)
      | end
  Out1 : Outport
  wires:
  In1/1 -> Out1/1

== system ES105A_StHlthSigNormn/StHlthSigNormn/UpdRawSig/Current Error/CurrMotSumDEFStHlth Calc/If Action Subsystem4/If Action Subsystem1/Divide by Zero Protection for Cal/CopyRight2 ==

== system ES105A_StHlthSigNormn/StHlthSigNormn/UpdRawSig/Current Error/CurrMotSumDEFStHlth Calc/If Action Subsystem4/If Action Subsystem1/Divide by Zero Protection for Cal/If Zero ==
  Action Port : ActionPort  ActionType=then
  Constant1 : Constant  Value=CURRMOTSUMDIVBYZEROPROTNVAL_AMPR_F32
  CopyRight2 : Subsystem  Description=|  mask(Copyright Information){none=on}
      | Copyright info block.                                               
      |                                                                     
      | Place copyright information at the top of every subsystem in design.
      mask prompts: none "No parameters"
      mask help: Place copyright information at the top of every subsystem in design.
      mask Display:
      | NxtrConf = 'Nexteer Confidential';
      | 
      | sys = bdroot; %handle for the current model ("system")
      | first = get_param(sys,'Created');
      | first = first(end-3:end);  %year is last four digits
      | 
      | last = get_param(sys,'LastModifiedDate');
      | if isempty(last)
      |     last = datestr(now,'yyyy');
      | else
      |     last = last(end-3:end);
      | end
      | 
      | if strcmp(first,last)
      |     fprintf('%s -- Copyright %s Nexteer',NxtrConf,first)
      | else
      |     fprintf('%s -- %s%s- %s Nexteer',NxtrConf,char(169),first,last)
      | end
  Out1 : Outport
  wires:
  Constant1/1 -> Out1/1

== system ES105A_StHlthSigNormn/StHlthSigNormn/UpdRawSig/Current Error/CurrMotSumDEFStHlth Calc/If Action Subsystem4/If Action Subsystem1/Divide by Zero Protection for Cal/Non Zero ==
  In1 : Inport
  Action Port : ActionPort  ActionType=else
  CopyRight2 : Subsystem  Description=|  mask(Copyright Information){none=on}
      | Copyright info block.                                               
      |                                                                     
      | Place copyright information at the top of every subsystem in design.
      mask prompts: none "No parameters"
      mask help: Place copyright information at the top of every subsystem in design.
      mask Display:
      | NxtrConf = 'Nexteer Confidential';
      | 
      | sys = bdroot; %handle for the current model ("system")
      | first = get_param(sys,'Created');
      | first = first(end-3:end);  %year is last four digits
      | 
      | last = get_param(sys,'LastModifiedDate');
      | if isempty(last)
      |     last = datestr(now,'yyyy');
      | else
      |     last = last(end-3:end);
      | end
      | 
      | if strcmp(first,last)
      |     fprintf('%s -- Copyright %s Nexteer',NxtrConf,first)
      | else
      |     fprintf('%s -- %s%s- %s Nexteer',NxtrConf,char(169),first,last)
      | end
  Out1 : Outport
  wires:
  In1/1 -> Out1/1

== system ES105A_StHlthSigNormn/StHlthSigNormn/UpdRawSig/Digital Torque Sensor /DigTqSnsrAStHlth Calc/If Action Subsystem1/Devide by Zero Protection for Cal/If Zero/CopyRight2 ==

== system ES105A_StHlthSigNormn/StHlthSigNormn/UpdRawSig/Digital Torque Sensor /DigTqSnsrAStHlth Calc/If Action Subsystem1/Devide by Zero Protection for Cal/Non Zero/CopyRight2 ==

== system ES105A_StHlthSigNormn/StHlthSigNormn/UpdRawSig/Digital Torque Sensor /DigTqSnsrBStHlth Calc/If Action Subsystem3/Devide by Zero Protection for Cal/If Zero/CopyRight2 ==

== system ES105A_StHlthSigNormn/StHlthSigNormn/UpdRawSig/Digital Torque Sensor /DigTqSnsrBStHlth Calc/If Action Subsystem3/Devide by Zero Protection for Cal/Non Zero/CopyRight2 ==

== system ES105A_StHlthSigNormn/StHlthSigNormn/UpdRawSig/Motor Position 2 /If Action Subsystem/If Action Subsystem1/Divide by Zero Protection for Cal/If Zero/CopyRight2 ==

== system ES105A_StHlthSigNormn/StHlthSigNormn/UpdRawSig/Motor Position 2 /If Action Subsystem/If Action Subsystem1/Divide by Zero Protection for Cal/Non Zero/CopyRight2 ==

== system ES105A_StHlthSigNormn/StHlthSigNormn/UpdRawSig/Motor Position 2 /If Action Subsystem/If Action Subsystem2/Divide by Zero Protection for Cal/If Zero/CopyRight2 ==

== system ES105A_StHlthSigNormn/StHlthSigNormn/UpdRawSig/Motor Position 2 /If Action Subsystem/If Action Subsystem2/Divide by Zero Protection for Cal/Non Zero/CopyRight2 ==

== system ES105A_StHlthSigNormn/StHlthSigNormn/UpdRawSig/Motor Position Error /AbsltMotPosABDifStHlth Calc/If Action Subsystem/If Action Subsystem1/Divide by Zero Protection for Cal/CopyRight2 ==

== system ES105A_StHlthSigNormn/StHlthSigNormn/UpdRawSig/Motor Position Error /AbsltMotPosABDifStHlth Calc/If Action Subsystem/If Action Subsystem1/Divide by Zero Protection for Cal/If Zero ==
  Action Port : ActionPort  ActionType=then
  Constant1 : Constant  Value=MOTPOSNERRDIVBYZEROPROTNVAL_MOTREV_U16
  CopyRight2 : Subsystem  Description=|  mask(Copyright Information){none=on}
      | Copyright info block.                                               
      |                                                                     
      | Place copyright information at the top of every subsystem in design.
      mask prompts: none "No parameters"
      mask help: Place copyright information at the top of every subsystem in design.
      mask Display:
      | NxtrConf = 'Nexteer Confidential';
      | 
      | sys = bdroot; %handle for the current model ("system")
      | first = get_param(sys,'Created');
      | first = first(end-3:end);  %year is last four digits
      | 
      | last = get_param(sys,'LastModifiedDate');
      | if isempty(last)
      |     last = datestr(now,'yyyy');
      | else
      |     last = last(end-3:end);
      | end
      | 
      | if strcmp(first,last)
      |     fprintf('%s -- Copyright %s Nexteer',NxtrConf,first)
      | else
      |     fprintf('%s -- %s%s- %s Nexteer',NxtrConf,char(169),first,last)
      | end
  Out1 : Outport
  wires:
  Constant1/1 -> Out1/1

== system ES105A_StHlthSigNormn/StHlthSigNormn/UpdRawSig/Motor Position Error /AbsltMotPosABDifStHlth Calc/If Action Subsystem/If Action Subsystem1/Divide by Zero Protection for Cal/Non Zero ==
  In1 : Inport
  Action Port : ActionPort  ActionType=else
  CopyRight2 : Subsystem  Description=|  mask(Copyright Information){none=on}
      | Copyright info block.                                               
      |                                                                     
      | Place copyright information at the top of every subsystem in design.
      mask prompts: none "No parameters"
      mask help: Place copyright information at the top of every subsystem in design.
      mask Display:
      | NxtrConf = 'Nexteer Confidential';
      | 
      | sys = bdroot; %handle for the current model ("system")
      | first = get_param(sys,'Created');
      | first = first(end-3:end);  %year is last four digits
      | 
      | last = get_param(sys,'LastModifiedDate');
      | if isempty(last)
      |     last = datestr(now,'yyyy');
      | else
      |     last = last(end-3:end);
      | end
      | 
      | if strcmp(first,last)
      |     fprintf('%s -- Copyright %s Nexteer',NxtrConf,first)
      | else
      |     fprintf('%s -- %s%s- %s Nexteer',NxtrConf,char(169),first,last)
      | end
  Out1 : Outport
  wires:
  In1/1 -> Out1/1

== system ES105A_StHlthSigNormn/StHlthSigNormn/UpdRawSig/Motor Position Error /AbsltMotPosACDifStHlth Calc/If Action Subsystem4/If Action Subsystem1/Divide by Zero Protection for Cal/CopyRight2 ==
